simulink model "Sensors"  (R2024a)
settings: Solver=VariableStepAuto  StartTime=0.0  StopTime=10.0  RelTol=1e-3
model workspace (MATLAB code in the model file):
  | SensorParams;
undefined symbols (not defined in the file): accelerometer_noise, gyro_noise
libraries: simulink x2
settings Model: Creator=Marij  LastModifiedBy=Marij
settings OptimizationCC: UseDivisionForNetSlopeComputation=on

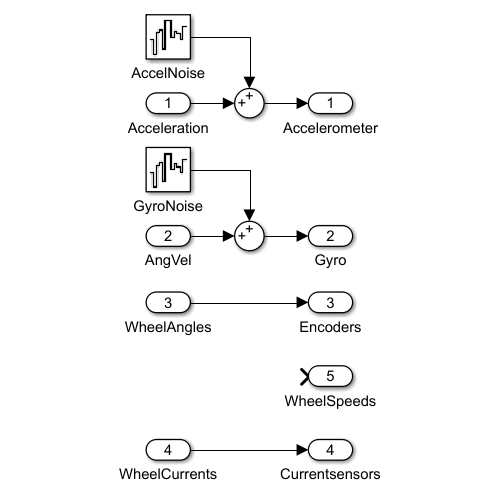
[thumbnail: Simulink's stored preview of the top-level diagram]
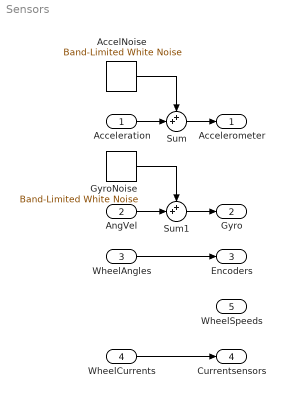
== system Sensors ==
  Acceleration : Inport  Unit=m/s^2  PortDimensions=2
  AngVel : Inport  Port=2  Unit=rad/s  PortDimensions=1
  WheelAngles : Inport  Port=3  Unit=rad  PortDimensions=4
  WheelCurrents : Inport  Port=4  Unit=A  PortDimensions=4
  AccelNoise : simulink/Sources/Band-Limited White Noise  Cov=[accelerometer_noise, accelerometer_noise]  Ts=0.01  seed=[23341]
  GyroNoise : simulink/Sources/Band-Limited White Noise  Cov=[gyro_noise]  Ts=0.01  seed=[23341]
  Sum : Sum  Inputs=++|
  Sum1 : Sum  Inputs=++|
  Accelerometer : Outport  Unit=m/s^2  PortDimensions=2
  Gyro : Outport  Port=2  Unit=rad/s  PortDimensions=1
  Encoders : Outport  Port=3  Unit=rad  PortDimensions=4
  Currentsensors : Outport  Port=4  Unit=A  PortDimensions=4
  WheelSpeeds : Outport  Port=5  Unit=rad/s  PortDimensions=4
  wires:
  Acceleration/1 -> Sum/2
  AccelNoise/1 -> Sum/1
  Sum/1 -> Accelerometer/1
  GyroNoise/1 -> Sum1/1
  Sum1/1 -> Gyro/1
  AngVel/1 -> Sum1/2
  WheelAngles/1 -> Encoders/1
  WheelCurrents/1 -> Currentsensors/1
